simulink model "verify_density_mdl_r2015b"  (R2015b)
settings: Solver=FixedStepDiscrete  StartTime=0.0  StopTime=1  FixedStep=1  RelTol=1e-3
values from neighbouring files (symbols this model uses):
  fmix = mix(n)    [verification_density.m]    (also in verification_fluidproperty.m; verification_heat_capacity.m; verification_kinematic_viscosity.m; verification_thermal_conductivity.m)
  press = p(m)    [verification_density.m]    (also in verification_fluidproperty.m; verification_heat_capacity.m; verification_kinematic_viscosity.m; verification_thermal_conductivity.m)
undefined symbols (not defined in the file or in its folder): fluid
libraries: carnot x1
settings Model: Creator=drhf  LastModifiedBy=drhf
settings DataIOCC: SaveFormat=Array  SignalLoggingSaveFormat=ModelDataLogs  SaveTime=off  ReturnWorkspaceOutputs=on  OutputSaveName=rho2
settings OptimizationCC: ExpressionDepthLimit=2147483647
settings DebuggingCC: UnderspecifiedInitializationDetection=Classic  MergeDetectMultiDrivingBlocksExec=none  SolverPrmCheckMsg=warning  FcnCallInpInsideContextMsg=UseLocalSettings  StateNameClashWarn=warning
settings HardwareCC: ProdBitPerPointer=32  ProdLargestAtomicFloat=None  ProdIntDivRoundTo=Undefined  ProdEndianess=Unspecified  ProdWordSize=32  ProdHWDeviceType=32-bit Generic
settings GRTTargetCC: GeneratePreprocessorConditionals=Disable all  CombineOutputUpdateFcns=off  GRTInterface=on
settings ConfigComp: CovModelRefEnable=Off

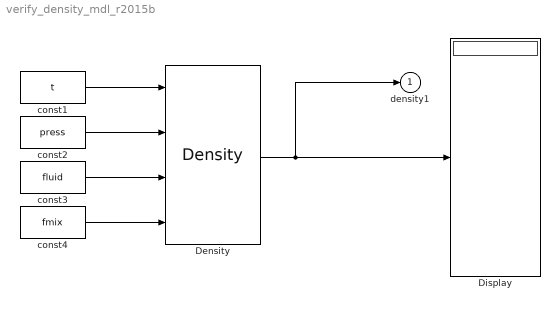
== system verify_density_mdl_r2015b ==
  Density : carnot/Basic/Material_Properties/Density  VariantControl=CarlibClassic  INPUTARGUMENTS=state variables (classic)  DEBUGLEVEL=DEBUGLEVEL  MAXTOTALWARNINGS=inf  MAXCONSECUTIVEWARNINGS=inf  WRITETOFILE=0  FILENAME='errors.txt'
  Display : Display
  const1 : Constant  Value=t
  const2 : Constant  Value=press
  const3 : Constant  Value=fluid
  const4 : Constant  Value=fmix
  density1 : Outport  InitialOutput=0
  wires:
  const2/1 -> Density/2
  const3/1 -> Density/3
  const4/1 -> Density/4
  const1/1 -> Density/1
  Density/1 -> Display/1, density1/1
